simulink model "Gear"  (R2021b)
settings: Solver=FixedStepDiscrete  StartTime=0.0  StopTime=10.0  FixedStep=0.001  RelTol=1e-3
libraries: simulink x1
settings Model: Creator=win  LastModifiedBy=win

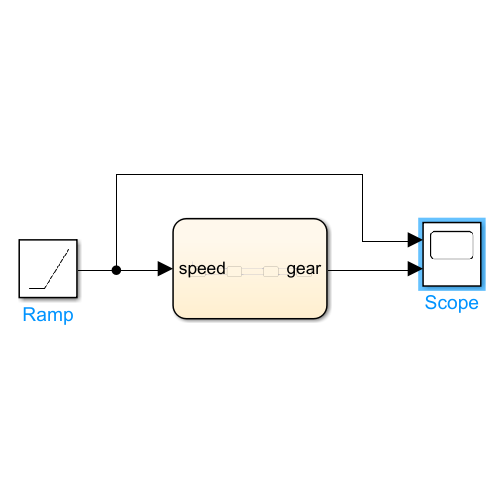
[thumbnail: Simulink's stored preview of the top-level diagram]
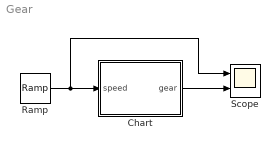
== system Gear ==
  Chart : Stateflow chart  TreatAsAtomicUnit=on
  Ramp : simulink/Sources/Ramp  slope=25  start=0  InitialOutput=0
  Scope : Scope  NumInputPorts=2
  wires:
  Ramp/1 -> Scope/1, Chart/1(speed)
  Chart/1(gear) -> Scope/2

== stateflow chart Gear/Chart ==
  state second
    during:
    gear = 2;
  state third
    during:
    gear = 3;
  state fourth
    during:
    gear = 4;
  state First
    during:
    gear = 1;
  (default) -> First
  second -> third [order 2] : [speed>50]
  third -> fourth [order 2] : [speed>100]
  First -> second : [speed>10]
  third -> second [order 1] : [speed<50]
  fourth -> third : [speed<100]
  second -> First [order 1] : [speed<10]
  data: speed input; gear output
